simulink model "Demo"  (Simulink 6.2)
settings: Solver=ode45  StartTime=0.0  StopTime=10.0  RelTol=1e-3
settings Model: Creator=suarezjl  LastModifiedBy=suarezjl
settings DataIOCC: SignalLoggingName=sigsOut
settings HardwareCC: TargetUnknown=on

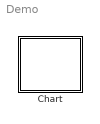
== system Demo ==
  Chart : Stateflow chart

== stateflow chart Chart ==
  state Start Cameras State Machine in Sally
    \\Sally\CogDemo\HeadModule\LeftCameraAgent\StateMachine.LoadSM()
    \\Sally\CogDemo\HeadModule\LeftCameraAgent\StateMachine.Start()
    \\Sally\CogDemo\HeadModule\RightCameraAgent\StateMachine.LoadSM()
    \\Sally\CogDemo\HeadModule\RightCameraAgent\StateMachine.Start()
  state Start Head
    \\Sally\CogDemo\HeadModule\HeadAgent\StateMachine.LoadSM()
    \\Sally\CogDemo\HeadModule\HeadAgent\StateMachine.Start()
  state Stop Head
    \\Sally\CogDemo\HeadModule\HeadAgent\StateMachine.Stop()
    \\Sally\CogDemo\HeadModule\LeftCameraAgent\StateMachine.Stop()
    \\Sally\CogDemo\HeadModule\RightCameraAgent\StateMachine.Stop()
    \\Hungerforce\CogDemo\RightArm\StateMachine.Stop()
    \\Hungerforce\CogDemo\RightTrajectoryAgent\StateMachine.Stop()
  state Start Arm and Trajectory Agent State Machines in Hungerforce
    \\Hungerforce\CogDemo\RightArm\StateMachine.LoadSM()
    \\Hungerforce\CogDemo\RightArm\StateMachine.Start()
    \\Hungerforce\CogDemo\RightTrajectoryAgent\StateMachine.LoadSM()
    \\Hungerforce\CogDemo\RightTrajectoryAgent\StateMachine.Start()
  (default) -> Start Cameras State Machine in Sally [order 1] : Start
  Start Cameras State Machine in Sally -> Start Head : Always
  (default) -> Start Arm and Trajectory Agent State Machines in Hungerforce [order 2] : Always
  Start Arm and Trajectory Agent State Machines in Hungerforce -> Stop Head : Signal="Stop"
